simulink model "second_order_DDPG"  (R2021a)
settings: Solver=VariableStepAuto  StartTime=0.0  StopTime=0.2  RelTol=1e-3
libraries: rllib x1, simulink x1
settings Model: Creator=Steven  LastModifiedBy=Steven

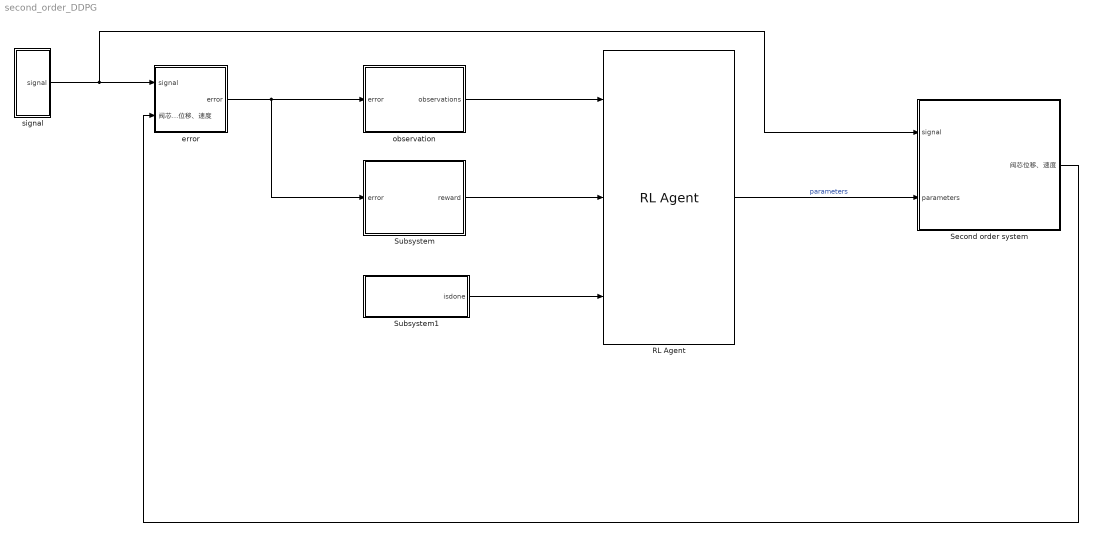
== system second_order_DDPG ==
  RL Agent : rllib/RL Agent  Agent=agent_second_order  ExternalActionAsInput=off  ProvideCumRwd=off  TreatAsDirectFeedthrough=on
  Second order system : Subsystem
  Subsystem : Subsystem
  Subsystem1 : Subsystem
  error : Subsystem
  observation : Subsystem
  signal : Subsystem
  wires:
  observation/1(observations) -> RL Agent/1
  RL Agent/1 -> Second order system/2(parameters)  "parameters"
  signal/1(signal) -> Second order system/1(signal), error/1(signal)
  Second order system/1(阀芯位移、速度) -> error/2(阀芯位移、速度)
  error/1(error) -> Subsystem/1(error), observation/1(error)
  Subsystem/1(reward) -> RL Agent/2
  Subsystem1/1(isdone) -> RL Agent/3

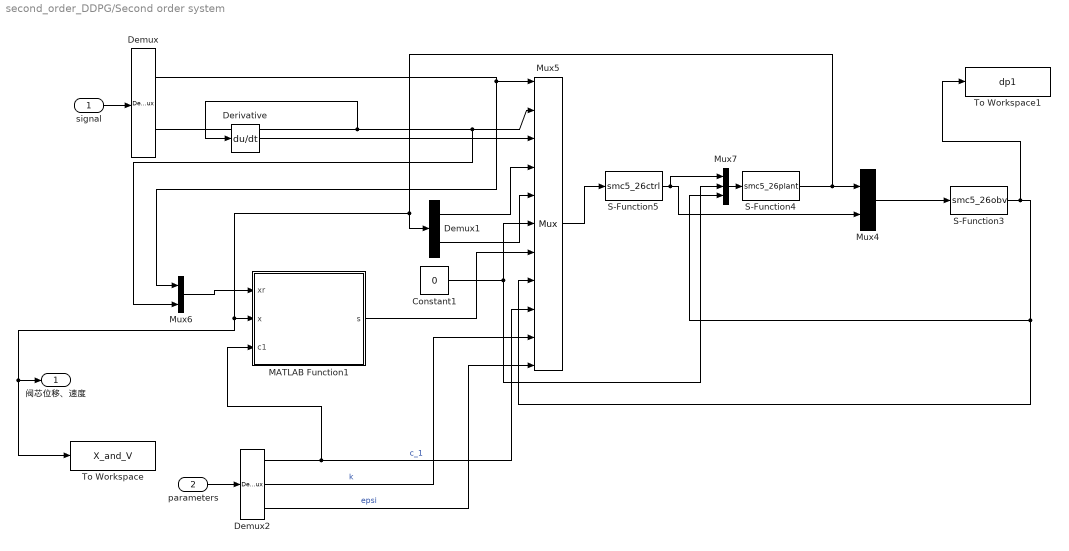
== system second_order_DDPG/Second order system ==
  signal : Inport
  parameters : Inport  Port=2
  Constant1 : Constant  Value=0
  Demux : Demux  Outputs=2
  Demux1 : Demux  Outputs=2
  Demux2 : Demux  Outputs=3
  Derivative : Derivative
  MATLAB Function1 : MATLAB Function  TreatAsAtomicUnit=on
  Mux4 : Mux  Inputs=2
  Mux5 : Mux  Inputs=11
  Mux6 : Mux  Inputs=2
  Mux7 : Mux  Inputs=3
  S-Function3 : S-Function  FunctionName=smc5_26obv  SFunctionDeploymentMode=off  EnableBusSupport=off
  S-Function4 : S-Function  FunctionName=smc5_26plant  SFunctionDeploymentMode=off  EnableBusSupport=off
  S-Function5 : S-Function  FunctionName=smc5_26ctrl  SFunctionDeploymentMode=off  EnableBusSupport=off
  To Workspace : ToWorkspace  VariableName=X_and_V  SampleTime=-1
      settings: Decimation=2
  To Workspace1 : ToWorkspace  VariableName=dp1  SampleTime=-1
      settings: Save2DSignal=2-D array (concatenate along first dimension)
  阀芯位移、速度 : Outport
  wires:
  S-Function3/1 -> To Workspace1/1, Mux7/3, Mux5/8
  Mux5/1 -> S-Function5/1
  Constant1/1 -> Mux7/2, Mux5/6
  MATLAB Function1/1(s) -> Mux5/7
  Demux1/2 -> Mux5/5
  S-Function4/1 -> Demux1/1, To Workspace/1, 阀芯位移、速度/1, MATLAB Function1/2(x), Mux4/1
  Mux4/1 -> S-Function3/1
  Mux6/1 -> MATLAB Function1/1(xr)
  Demux/1 -> Mux6/1, Mux5/1
  Demux1/1 -> Mux5/4
  Mux7/1 -> S-Function4/1
  S-Function5/1 -> Mux7/1, Mux4/2
  signal/1 -> Demux/1
  Demux/2 -> Mux6/2, Mux5/2, Derivative/1
  parameters/1 -> Demux2/1
  Demux2/1 -> MATLAB Function1/3(c1), Mux5/9  "c_1"
  Demux2/2 -> Mux5/10  "k"
  Demux2/3 -> Mux5/11  "epsi"
  Derivative/1 -> Mux5/3

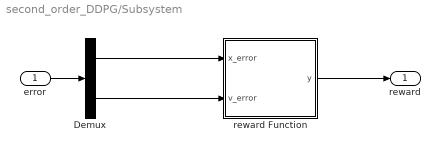
== system second_order_DDPG/Subsystem ==
  error : Inport
  Demux : Demux  Outputs=2
  reward Function : MATLAB Function  TreatAsAtomicUnit=on
  reward : Outport
  wires:
  error/1 -> Demux/1
  Demux/1 -> reward Function/1(x_error)
  Demux/2 -> reward Function/2(v_error)
  reward Function/1(y) -> reward/1

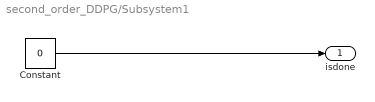
== system second_order_DDPG/Subsystem1 ==
  Constant : Constant  Value=0
  isdone : Outport
  wires:
  Constant/1 -> isdone/1

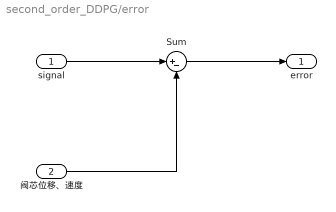
== system second_order_DDPG/error ==
  signal : Inport
  阀芯位移、速度 : Inport  Port=2
  Sum : Sum  Inputs=|+-
  error : Outport
  wires:
  signal/1 -> Sum/1
  阀芯位移、速度/1 -> Sum/2
  Sum/1 -> error/1

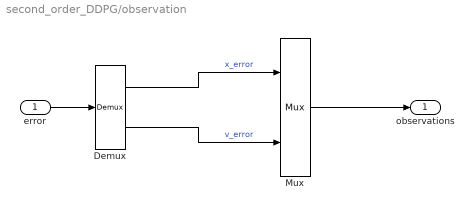
== system second_order_DDPG/observation ==
  error : Inport
  Demux : Demux  Outputs=2
  Mux : Mux  Inputs=2
  observations : Outport
  wires:
  Mux/1 -> observations/1
  error/1 -> Demux/1
  Demux/1 -> Mux/1  "x_error"
  Demux/2 -> Mux/2  "v_error"

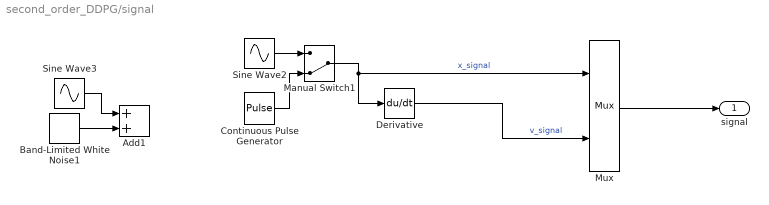
== system second_order_DDPG/signal ==
  Add1 : Sum
  Band-Limited White Noise1 : simulink/Sources/Band-Limited White Noise  Cov=[1e-5*1e-5*0.1]  Ts=0.1  seed=[0]
  Continuous Pulse Generator : DiscretePulseGenerator  PulseType=Time based  Amplitude=1e-4  Period=0.2  PulseWidth=50
  Derivative : Derivative
  Manual Switch1 : ManualSwitch  CurrentSetting=0
  Mux : Mux  Inputs=2
  Sine Wave2 : Sin  Amplitude=1e-3  Frequency=20*pi  SampleTime=0
  Sine Wave3 : Sin  Amplitude=1e-4  Frequency=30*pi  SampleTime=0
  signal : Outport
  wires:
  Sine Wave2/1 -> Manual Switch1/1
  Continuous Pulse Generator/1 -> Manual Switch1/2
  Manual Switch1/1 -> Mux/1, Derivative/1  "x_signal"
  Derivative/1 -> Mux/2  "v_signal"
  Mux/1 -> signal/1
  Band-Limited White Noise1/1 -> Add1/2
  Sine Wave3/1 -> Add1/1

== matlab function second_order_DDPG/Subsystem/reward Function ==
  data: x_error input; y output; v_error input
function y = fcn(x_error,v_error)
y = -x_error^2*2.5e5;

== matlab function second_order_DDPG/Second order system/MATLAB Function1 ==
  data: xr input; s output; x input; c1 input
function s = S(xr,x,c1)
s = c1*(xr(1)-x(1)) + (xr(2)-x(2));
